simulink model "simulink_model_parteB_random"  (R2023b)
settings: Solver=VariableStepAuto  StartTime=0.0  StopTime=10  RelTol=1e-3
settings Model: Creator=jbsantos  LastModifiedBy=jbsantos

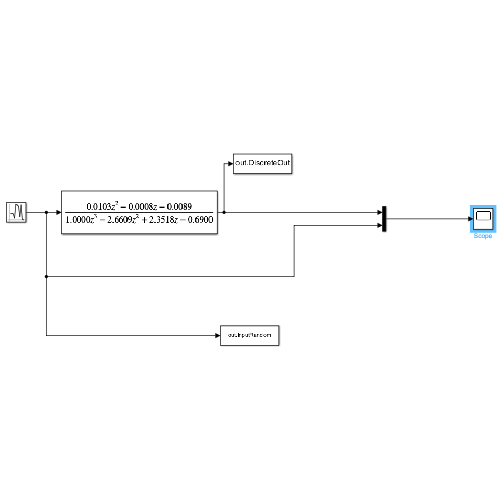
[thumbnail: Simulink's stored preview of the top-level diagram]
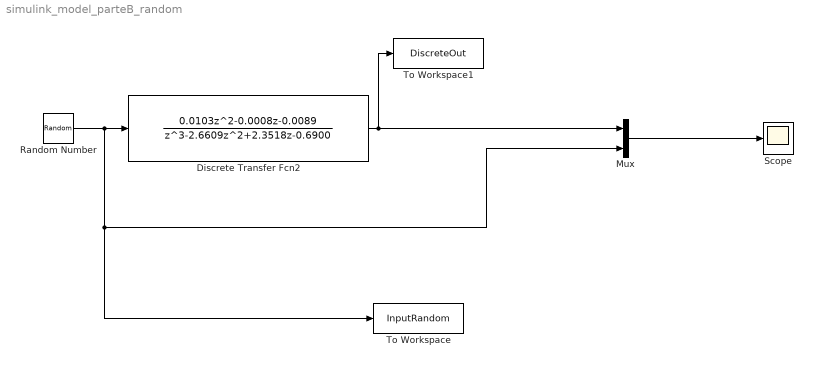
== system simulink_model_parteB_random ==
  Discrete Transfer Fcn2 : DiscreteTransferFcn  Numerator="[0    0.0103   -0.0008   -0.0089]"  Denominator="[1.0000   -2.6609    2.3518   -0.6900]"
  Mux : Mux  Inputs=2
  Random Number : RandomNumber  SampleTime=0.1
  Scope : Scope
  To Workspace : ToWorkspace  VariableName=InputRandom  SaveFormat=Timeseries  SampleTime=-1
  To Workspace1 : ToWorkspace  VariableName=DiscreteOut  SaveFormat=Timeseries  SampleTime=-1
  wires:
  Random Number/1 -> Discrete Transfer Fcn2/1, To Workspace/1, Mux/2
  Discrete Transfer Fcn2/1 -> To Workspace1/1, Mux/1
  Mux/1 -> Scope/1
